simulink model "SoftManipulatorModel"  (R2019a)
settings: Solver=VariableStepAuto  StartTime=0.0  StopTime=100  FixedStep=0.01  RelTol=1e-3
undefined symbols (not defined in the file): d, dq_init, k, l, m, q_init
libraries: dspinverses x1
(part 2 of 2)

== matlab function SoftManipulatorModel/Controller/Coriolis Matrix ==
  data: q input; Cq output; dq input; m input; l input
function Cq = fcn(q, dq, m, l)

q1 = q(1);
q2 = q(2);
dq1 = dq(1);
dq2 = dq(2);
m1 = m(1);
m2 = m(2);
l1 = l(1);
l2 = l(2);

Cq = zeros(2,2);
% C111 = 0;
% C121 = 0;
% C221 = 0;
% C112 = 0;
% C222 = 0;
% tolerance = 1e-3;
% fake_zero = 1e-3;

% This equation got from Matlab symbolic calculation
% if abs(q1) < tolerance && abs(q2) > tolerance
%     C111 = 0;
%     C121 = -(m2*((l2*sin(conj(q2))*conj(l2)*(cos(q2) - 1))/(4*q2*conj(q2)) - ((l2*cos(q2))/(2*q2) - (l2*sin(q2))/(2*q2^2))*(conj(l1) + (sin(conj(q2))*conj(l2))/(2*conj(q2))) - (l1 + (l2*sin(q2))/(2*q2))*((cos(conj(q2))*conj(l2))/(2*conj(q2)) - (sin(conj(q2))*conj(l2))/(2*conj(q2)^2)) + (l2*conj(l2)*sin(q2)*(cos(conj(q2)) - 1))/(4*q2*conj(q2)) + (l2*conj(l2)*(cos(q2) - 1)*(cos(conj(q2)) - 1))/(4*q2*conj(q2)^2) + (l2*conj(l2)*(cos(q2) - 1)*(cos(conj(q2)) - 1))/(4*q2^2*conj(q2))))/2;
%     C221 = -m2*((l2*sin(q2)*(conj(l1) + (sin(conj(q2))*conj(l2))/(2*conj(q2))))/(2*q2^2) - (l2*cos(q2)*(conj(l1) + (sin(conj(q2))*conj(l2))/(2*conj(q2))))/(2*q2) - (l2*sin(q2)*((cos(conj(q2))*conj(l2))/(2*conj(q2)) - (sin(conj(q2))*conj(l2))/(2*conj(q2)^2)))/(2*q2) + (l2*sin(conj(q2))*conj(l2)*(cos(q2) - 1))/(4*q2*conj(q2)) + (l2*conj(l2)*sin(q2)*(cos(conj(q2)) - 1))/(4*q2*conj(q2)) + (l2*conj(l2)*(cos(q2) - 1)*(cos(conj(q2)) - 1))/(4*q2*conj(q2)^2) + (l2*conj(l2)*(cos(q2) - 1)*(cos(conj(q2)) - 1))/(4*q2^2*conj(q2)));
%     C112 = (m2*((l2*sin(conj(q2))*conj(l2)*(cos(q2) - 1))/(4*q2*conj(q2)) - ((l2*cos(q2))/(2*q2) - (l2*sin(q2))/(2*q2^2))*(conj(l1) + (sin(conj(q2))*conj(l2))/(2*conj(q2))) - (l1 + (l2*sin(q2))/(2*q2))*((cos(conj(q2))*conj(l2))/(2*conj(q2)) - (sin(conj(q2))*conj(l2))/(2*conj(q2)^2)) + (l2*conj(l2)*sin(q2)*(cos(conj(q2)) - 1))/(4*q2*conj(q2)) + (l2*conj(l2)*(cos(q2) - 1)*(cos(conj(q2)) - 1))/(4*q2*conj(q2)^2) + (l2*conj(l2)*(cos(q2) - 1)*(cos(conj(q2)) - 1))/(4*q2^2*conj(q2))))/2;
%     C222 = -(m2*((l2*sin(conj(q2))*conj(l2)*(cos(q2) - 1))/(4*q2*conj(q2)) + (l2*conj(l2)*sin(q2)*(cos(conj(q2)) - 1))/(4*q2*conj(q2)) + (l2*conj(l2)*(cos(q2) - 1)*(cos(conj(q2)) - 1))/(4*q2*conj(q2)^2) + (l2*conj(l2)*(cos(q2) - 1)*(cos(conj(q2)) - 1))/(4*q2^2*conj(q2)) - (l2*cos(conj(q2))*conj(l2)*sin(q2))/(4*q2*conj(q2)) - (l2*sin(conj(q2))*conj(l2)*cos(q2))/(4*q2*conj(q2)) + (l2*sin(conj(q2))*conj(l2)*sin(q2))/(4*q2*conj(q2)^2) + (l2*sin(conj(q2))*conj(l2)*sin(q2))/(4*q2^2*conj(q2))))/2;
% elseif abs(q1) < tolerance && abs(q2) < tolerance
%     C111 = 0;
%     C121 = 0;
%     C221 = 0;
%     C112 = 0;
%     C222 = 0;
% elseif abs(q1) > tolerance && abs(q2) < tolerance
%     C111 = m2*(((sin(conj(q1))*conj(l2))/2 - (conj(l1)*(cos(conj(q1)) - 1))/conj(q1))*((l2*cos(q1))/2 + (l1*sin(q1))/q1 + (l1*(cos(q1) - 1))/q1^2) + ((l2*sin(q1))/2 - (l1*(cos(q1) - 1))/q1)*((cos(conj(q1))*conj(l2))/2 + (sin(conj(q1))*conj(l1))/conj(q1) + (conj(l1)*(cos(conj(q1)) - 1))/conj(q1)^2) - ((cos(conj(q1))*conj(l2))/2 + (sin(conj(q1))*conj(l1))/conj(q1))*((l2*sin(q1))/2 - (l1*cos(q1))/q1 + (l1*sin(q1))/q1^2) - ((l2*cos(q1))/2 + (l1*sin(q1))/q1)*((sin(conj(q1))*conj(l2))/2 - (cos(conj(q1))*conj(l1))/conj(q1) + (sin(conj(q1))*conj(l1))/conj(q1)^2)) - m1*((l1*sin(conj(q1))*conj(l1)*(cos(q1) - 1))/(4*q1*conj(q1)) + (l1*conj(l1)*sin(q1)*(cos(conj(q1)) - 1))/(4*q1*conj(q1)) + (l1*conj(l1)*(cos(q1) - 1)*(cos(conj(q1)) - 1))/(4*q1*conj(q1)^2) + (l1*conj(l1)*(cos(q1) - 1)*(cos(conj(q1)) - 1))/(4*q1^2*conj(q1)) - (l1*cos(conj(q1))*conj(l1)*sin(q1))/(4*q1*conj(q1)) - (l1*sin(conj(q1))*conj(l1)*cos(q1))/(4*q1*conj(q1)) + (l1*sin(conj(q1))*conj(l1)*sin(q1))/(4*q1*conj(q1)^2) + (l1*sin(conj(q1))*conj(l1)*sin(q1))/(4*q1^2*conj(q1)));
%     C121 = 0;
%     C221 = 0;
%     C112 = m2*((cos(conj(q1))*conj(l2)*((l2*sin(q1))/2 - (l1*(cos(q1) - 1))/q1))/2 - (cos(conj(q1))*conj(l2)*((l2*sin(q1))/2 - (l1*cos(q1))/q1 + (l1*sin(q1))/q1^2))/2 + (sin(conj(q1))*conj(l2)*((l2*cos(q1))/2 + (l1*sin(q1))/q1 + (l1*(cos(q1) - 1))/q1^2))/2 - (sin(conj(q1))*conj(l2)*((l2*cos(q1))/2 + (l1*sin(q1))/q1))/2);
%     C222 = 0;
% elseif abs(q1) > tolerance && abs(q2) > tolerance
%     C111 = m2*(((l1*sin(q1))/q1 + (l2*cos(q1)*sin(q2))/(2*q2) + (l2*sin(q1)*(cos(q2) - 1))/(2*q2))*((cos(conj(q1))*conj(l1))/conj(q1) - (sin(conj(q1))*conj(l1))/conj(q1)^2 + (cos(conj(q1))*conj(l2)*(cos(conj(q2)) - 1))/(2*conj(q2)) - (sin(conj(q1))*sin(conj(q2))*conj(l2))/(2*conj(q2))) - ((conj(l1)*(cos(conj(q1)) - 1))/conj(q1) + (cos(conj(q1))*conj(l2)*(cos(conj(q2)) - 1))/(2*conj(q2)) - (sin(conj(q1))*sin(conj(q2))*conj(l2))/(2*conj(q2)))*((l1*sin(q1))/q1 + (l1*(cos(q1) - 1))/q1^2 + (l2*cos(q1)*sin(q2))/(2*q2) + (l2*sin(q1)*(cos(q2) - 1))/(2*q2)) - ((l1*(cos(q1) - 1))/q1 - (l2*sin(q1)*sin(q2))/(2*q2) + (l2*cos(q1)*(cos(q2) - 1))/(2*q2))*((sin(conj(q1))*conj(l1))/conj(q1) + (conj(l1)*(cos(conj(q1)) - 1))/conj(q1)^2 + (sin(conj(q1))*conj(l2)*(cos(conj(q2)) - 1))/(2*conj(q2)) + (cos(conj(q1))*sin(conj(q2))*conj(l2))/(2*conj(q2))) + ((sin(conj(q1))*conj(l1))/conj(q1) + (sin(conj(q1))*conj(l2)*(cos(conj(q2)) - 1))/(2*conj(q2)) + (cos(conj(q1))*sin(conj(q2))*conj(l2))/(2*conj(q2)))*((l1*cos(q1))/q1 - (l1*sin(q1))/q1^2 - (l2*sin(q1)*sin(q2))/(2*q2) + (l2*cos(q1)*(cos(q2) - 1))/(2*q2))) - m1*((l1*sin(conj(q1))*conj(l1)*(cos(q1) - 1))/(4*q1*conj(q1)) + (l1*conj(l1)*sin(q1)*(cos(conj(q1)) - 1))/(4*q1*conj(q1)) + (l1*conj(l1)*(cos(q1) - 1)*(cos(conj(q1)) - 1))/(4*q1*conj(q1)^2) + (l1*conj(l1)*(cos(q1) - 1)*(cos(conj(q1)) - 1))/(4*q1^2*conj(q1)) - (l1*cos(conj(q1))*conj(l1)*sin(q1))/(4*q1*conj(q1)) - (l1*sin(conj(q1))*conj(l1)*cos(q1))/(4*q1*conj(q1)) + (l1*sin(conj(q1))*conj(l1)*sin(q1))/(4*q1*conj(q1)^2) + (l1*sin(conj(q1))*conj(l1)*sin(q1))/(4*q1^2*conj(q1)));
%     C121 = -(m2*(((l1*sin(q1))/q1 + (l2*cos(q1)*sin(q2))/(2*q2) + (l2*sin(q1)*(cos(q2) - 1))/(2*q2))*((sin(conj(q1))*conj(l2)*(cos(conj(q2)) - 1))/(2*conj(q2)^2) - (cos(conj(q1))*cos(conj(q2))*conj(l2))/(2*conj(q2)) + (cos(conj(q1))*sin(conj(q2))*conj(l2))/(2*conj(q2)^2) + (sin(conj(q1))*sin(conj(q2))*conj(l2))/(2*conj(q2))) + ((sin(conj(q1))*conj(l1))/conj(q1) + (sin(conj(q1))*conj(l2)*(cos(conj(q2)) - 1))/(2*conj(q2)) + (cos(conj(q1))*sin(conj(q2))*conj(l2))/(2*conj(q2)))*((l2*cos(q1)*sin(q2))/(2*q2^2) - (l2*cos(q1)*cos(q2))/(2*q2) + (l2*sin(q1)*sin(q2))/(2*q2) + (l2*sin(q1)*(cos(q2) - 1))/(2*q2^2)) + ((l1*(cos(q1) - 1))/q1 - (l2*sin(q1)*sin(q2))/(2*q2) + (l2*cos(q1)*(cos(q2) - 1))/(2*q2))*((cos(conj(q1))*conj(l2)*(cos(conj(q2)) - 1))/(2*conj(q2)^2) + (cos(conj(q1))*sin(conj(q2))*conj(l2))/(2*conj(q2)) + (cos(conj(q2))*sin(conj(q1))*conj(l2))/(2*conj(q2)) - (sin(conj(q1))*sin(conj(q2))*conj(l2))/(2*conj(q2)^2)) + ((conj(l1)*(cos(conj(q1)) - 1))/conj(q1) + (cos(conj(q1))*conj(l2)*(cos(conj(q2)) - 1))/(2*conj(q2)) - (sin(conj(q1))*sin(conj(q2))*conj(l2))/(2*conj(q2)))*((l2*cos(q1)*sin(q2))/(2*q2) + (l2*cos(q2)*sin(q1))/(2*q2) - (l2*sin(q1)*sin(q2))/(2*q2^2) + (l2*cos(q1)*(cos(q2) - 1))/(2*q2^2))))/2;
%     C221 = -m2*(((l2*cos(q1)*sin(q2))/(2*q2) + (l2*sin(q1)*(cos(q2) - 1))/(2*q2))*((sin(conj(q1))*conj(l2)*(cos(conj(q2)) - 1))/(2*conj(q2)^2) - (cos(conj(q1))*cos(conj(q2))*conj(l2))/(2*conj(q2)) + (cos(conj(q1))*sin(conj(q2))*conj(l2))/(2*conj(q2)^2) + (sin(conj(q1))*sin(conj(q2))*conj(l2))/(2*conj(q2))) - ((l2*sin(q1)*sin(q2))/(2*q2) - (l2*cos(q1)*(cos(q2) - 1))/(2*q2))*((cos(conj(q1))*conj(l2)*(cos(conj(q2)) - 1))/(2*conj(q2)^2) + (cos(conj(q1))*sin(conj(q2))*conj(l2))/(2*conj(q2)) + (cos(conj(q2))*sin(conj(q1))*conj(l2))/(2*conj(q2)) - (sin(conj(q1))*sin(conj(q2))*conj(l2))/(2*conj(q2)^2)) + ((sin(conj(q1))*conj(l1))/conj(q1) + (sin(conj(q1))*conj(l2)*(cos(conj(q2)) - 1))/(2*conj(q2)) + (cos(conj(q1))*sin(conj(q2))*conj(l2))/(2*conj(q2)))*((l2*cos(q1)*sin(q2))/(2*q2^2) - (l2*cos(q1)*cos(q2))/(2*q2) + (l2*sin(q1)*sin(q2))/(2*q2) + (l2*sin(q1)*(cos(q2) - 1))/(2*q2^2)) + ((conj(l1)*(cos(conj(q1)) - 1))/conj(q1) + (cos(conj(q1))*conj(l2)*(cos(conj(q2)) - 1))/(2*conj(q2)) - (sin(conj(q1))*sin(conj(q2))*conj(l2))/(2*conj(q2)))*((l2*cos(q1)*sin(q2))/(2*q2) + (l2*cos(q2)*sin(q1))/(2*q2) - (l2*sin(q1)*sin(q2))/(2*q2^2) + (l2*cos(q1)*(cos(q2) - 1))/(2*q2^2)));
%     C112 = (m2*(((l1*sin(q1))/q1 + (l2*cos(q1)*sin(q2))/(2*q2) + (l2*sin(q1)*(cos(q2) - 1))/(2*q2))*((sin(conj(q1))*conj(l2)*(cos(conj(q2)) - 1))/(2*conj(q2)^2) - (cos(conj(q1))*cos(conj(q2))*conj(l2))/(2*conj(q2)) + (cos(conj(q1))*sin(conj(q2))*conj(l2))/(2*conj(q2)^2) + (sin(conj(q1))*sin(conj(q2))*conj(l2))/(2*conj(q2))) + ((sin(conj(q1))*conj(l1))/conj(q1) + (sin(conj(q1))*conj(l2)*(cos(conj(q2)) - 1))/(2*conj(q2)) + (cos(conj(q1))*sin(conj(q2))*conj(l2))/(2*conj(q2)))*((l2*cos(q1)*sin(q2))/(2*q2^2) - (l2*cos(q1)*cos(q2))/(2*q2) + (l2*sin(q1)*sin(q2))/(2*q2) + (l2*sin(q1)*(cos(q2) - 1))/(2*q2^2)) + ((l1*(cos(q1) - 1))/q1 - (l2*sin(q1)*sin(q2))/(2*q2) + (l2*cos(q1)*(cos(q2) - 1))/(2*q2))*((cos(conj(q1))*conj(l2)*(cos(conj(q2)) - 1))/(2*conj(q2)^2) + (cos(conj(q1))*sin(conj(q2))*conj(l2))/(2*conj(q2)) + (cos(conj(q2))*sin(conj(q1))*conj(l2))/(2*conj(q2)) - (sin(conj(q1))*sin(conj(q2))*conj(l2))/(2*conj(q2)^2)) + ((conj(l1)*(cos(conj(q1)) - 1))/conj(q1) + (cos(conj(q1))*conj(l2)*(cos(conj(q2)) - 1))/(2*conj(q2)) - (sin(conj(q1))*sin(conj(q2))*conj(l2))/(2*conj(q2)))*((l2*cos(q1)*sin(q2))/(2*q2) + (l2*cos(q2)*sin(q1))/(2*q2) - (l2*sin(q1)*sin(q2))/(2*q2^2) + (l2*cos(q1)*(cos(q2) - 1))/(2*q2^2))))/2 - m2*(((sin(conj(q1))*conj(l2)*(cos(conj(q2)) - 1))/(2*conj(q2)) + (cos(conj(q1))*sin(conj(q2))*conj(l2))/(2*conj(q2)))*((l1*(cos(q1) - 1))/q1 - (l2*sin(q1)*sin(q2))/(2*q2) + (l2*cos(q1)*(cos(q2) - 1))/(2*q2)) - ((sin(conj(q1))*conj(l2)*(cos(conj(q2)) - 1))/(2*conj(q2)) + (cos(conj(q1))*sin(conj(q2))*conj(l2))/(2*conj(q2)))*((l1*cos(q1))/q1 - (l1*sin(q1))/q1^2 - (l2*sin(q1)*sin(q2))/(2*q2) + (l2*cos(q1)*(cos(q2) - 1))/(2*q2)) + ((cos(conj(q1))*conj(l2)*(cos(conj(q2)) - 1))/(2*conj(q2)) - (sin(conj(q1))*sin(conj(q2))*conj(l2))/(2*conj(q2)))*((l1*sin(q1))/q1 + (l1*(cos(q1) - 1))/q1^2 + (l2*cos(q1)*sin(q2))/(2*q2) + (l2*sin(q1)*(cos(q2) - 1))/(2*q2)) - ((cos(conj(q1))*conj(l2)*(cos(conj(q2)) - 1))/(2*conj(q2)) - (sin(conj(q1))*sin(conj(q2))*conj(l2))/(2*conj(q2)))*((l1*sin(q1))/q1 + (l2*cos(q1)*sin(q2))/(2*q2) + (l2*sin(q1)*(cos(q2) - 1))/(2*q2)));
%     C222 = -(m2*(((l2*cos(q1)*sin(q2))/(2*q2) + (l2*sin(q1)*(cos(q2) - 1))/(2*q2))*((sin(conj(q1))*conj(l2)*(cos(conj(q2)) - 1))/(2*conj(q2)^2) - (cos(conj(q1))*cos(conj(q2))*conj(l2))/(2*conj(q2)) + (cos(conj(q1))*sin(conj(q2))*conj(l2))/(2*conj(q2)^2) + (sin(conj(q1))*sin(conj(q2))*conj(l2))/(2*conj(q2))) - ((l2*sin(q1)*sin(q2))/(2*q2) - (l2*cos(q1)*(cos(q2) - 1))/(2*q2))*((cos(conj(q1))*conj(l2)*(cos(conj(q2)) - 1))/(2*conj(q2)^2) + (cos(conj(q1))*sin(conj(q2))*conj(l2))/(2*conj(q2)) + (cos(conj(q2))*sin(conj(q1))*conj(l2))/(2*conj(q2)) - (sin(conj(q1))*sin(conj(q2))*conj(l2))/(2*conj(q2)^2)) + ((cos(conj(q1))*conj(l2)*(cos(conj(q2)) - 1))/(2*conj(q2)) - (sin(conj(q1))*sin(conj(q2))*conj(l2))/(2*conj(q2)))*((l2*cos(q1)*sin(q2))/(2*q2) + (l2*cos(q2)*sin(q1))/(2*q2) - (l2*sin(q1)*sin(q2))/(2*q2^2) + (l2*cos(q1)*(cos(q2) - 1))/(2*q2^2)) + ((sin(conj(q1))*conj(l2)*(cos(conj(q2)) - 1))/(2*conj(q2)) + (cos(conj(q1))*sin(conj(q2))*conj(l2))/(2*conj(q2)))*((l2*cos(q1)*sin(q2))/(2*q2^2) - (l2*cos(q1)*cos(q2))/(2*q2) + (l2*sin(q1)*sin(q2))/(2*q2) + (l2*sin(q1)*(cos(q2) - 1))/(2*q2^2))))/2;
% end

% if abs(q1) < tolerance && abs(q2) > tolerance
%     if q1 < 0
%         q1 = -fake_zero;
%     else
%         q1 = fake_zero;
%     end
% elseif abs(q1) < tolerance && abs(q2) < tolerance
%     if q1 < 0
%         q1 = -fake_zero;
%     else
%         q1 = fake_zero;
%     end
%     
%     if q2 < 0
%         q2 = -fake_zero;
%     else
%         q2 = fake_zero;
%     end
% elseif abs(q1) > tolerance && abs(q2) < tolerance
%     if q2 < 0
%         q2 = -fake_zero;
%     else
%         q2 = fake_zero;
%     end
% end

C111 = m2*(((l1*sin(q1))/q1 + (l2*cos(q1)*sin(q2))/(2*q2) + (l2*sin(q1)*(cos(q2) - 1))/(2*q2))*((cos(conj(q1))*conj(l1))/conj(q1) - (sin(conj(q1))*conj(l1))/conj(q1)^2 + (cos(conj(q1))*conj(l2)*(cos(conj(q2)) - 1))/(2*conj(q2)) - (sin(conj(q1))*sin(conj(q2))*conj(l2))/(2*conj(q2))) - ((conj(l1)*(cos(conj(q1)) - 1))/conj(q1) + (cos(conj(q1))*conj(l2)*(cos(conj(q2)) - 1))/(2*conj(q2)) - (sin(conj(q1))*sin(conj(q2))*conj(l2))/(2*conj(q2)))*((l1*sin(q1))/q1 + (l1*(cos(q1) - 1))/q1^2 + (l2*cos(q1)*sin(q2))/(2*q2) + (l2*sin(q1)*(cos(q2) - 1))/(2*q2)) - ((l1*(cos(q1) - 1))/q1 - (l2*sin(q1)*sin(q2))/(2*q2) + (l2*cos(q1)*(cos(q2) - 1))/(2*q2))*((sin(conj(q1))*conj(l1))/conj(q1) + (conj(l1)*(cos(conj(q1)) - 1))/conj(q1)^2 + (sin(conj(q1))*conj(l2)*(cos(conj(q2)) - 1))/(2*conj(q2)) + (cos(conj(q1))*sin(conj(q2))*conj(l2))/(2*conj(q2))) + ((sin(conj(q1))*conj(l1))/conj(q1) + (sin(conj(q1))*conj(l2)*(cos(conj(q2)) - 1))/(2*conj(q2)) + (cos(conj(q1))*sin(conj(q2))*conj(l2))/(2*conj(q2)))*((l1*cos(q1))/q1 - (l1*sin(q1))/q1^2 - (l2*sin(q1)*sin(q2))/(2*q2) + (l2*cos(q1)*(cos(q2) - 1))/(2*q2))) - m1*((l1*sin(conj(q1))*conj(l1)*(cos(q1) - 1))/(4*q1*conj(q1)) + (l1*conj(l1)*sin(q1)*(cos(conj(q1)) - 1))/(4*q1*conj(q1)) + (l1*conj(l1)*(cos(q1) - 1)*(cos(conj(q1)) - 1))/(4*q1*conj(q1)^2) + (l1*conj(l1)*(cos(q1) - 1)*(cos(conj(q1)) - 1))/(4*q1^2*conj(q1)) - (l1*cos(conj(q1))*conj(l1)*sin(q1))/(4*q1*conj(q1)) - (l1*sin(conj(q1))*conj(l1)*cos(q1))/(4*q1*conj(q1)) + (l1*sin(conj(q1))*conj(l1)*sin(q1))/(4*q1*conj(q1)^2) + (l1*sin(conj(q1))*conj(l1)*sin(q1))/(4*q1^2*conj(q1)));
C121 = -(m2*(((l1*sin(q1))/q1 + (l2*cos(q1)*sin(q2))/(2*q2) + (l2*sin(q1)*(cos(q2) - 1))/(2*q2))*((sin(conj(q1))*conj(l2)*(cos(conj(q2)) - 1))/(2*conj(q2)^2) - (cos(conj(q1))*cos(conj(q2))*conj(l2))/(2*conj(q2)) + (cos(conj(q1))*sin(conj(q2))*conj(l2))/(2*conj(q2)^2) + (sin(conj(q1))*sin(conj(q2))*conj(l2))/(2*conj(q2))) + ((sin(conj(q1))*conj(l1))/conj(q1) + (sin(conj(q1))*conj(l2)*(cos(conj(q2)) - 1))/(2*conj(q2)) + (cos(conj(q1))*sin(conj(q2))*conj(l2))/(2*conj(q2)))*((l2*cos(q1)*sin(q2))/(2*q2^2) - (l2*cos(q1)*cos(q2))/(2*q2) + (l2*sin(q1)*sin(q2))/(2*q2) + (l2*sin(q1)*(cos(q2) - 1))/(2*q2^2)) + ((l1*(cos(q1) - 1))/q1 - (l2*sin(q1)*sin(q2))/(2*q2) + (l2*cos(q1)*(cos(q2) - 1))/(2*q2))*((cos(conj(q1))*conj(l2)*(cos(conj(q2)) - 1))/(2*conj(q2)^2) + (cos(conj(q1))*sin(conj(q2))*conj(l2))/(2*conj(q2)) + (cos(conj(q2))*sin(conj(q1))*conj(l2))/(2*conj(q2)) - (sin(conj(q1))*sin(conj(q2))*conj(l2))/(2*conj(q2)^2)) + ((conj(l1)*(cos(conj(q1)) - 1))/conj(q1) + (cos(conj(q1))*conj(l2)*(cos(conj(q2)) - 1))/(2*conj(q2)) - (sin(conj(q1))*sin(conj(q2))*conj(l2))/(2*conj(q2)))*((l2*cos(q1)*sin(q2))/(2*q2) + (l2*cos(q2)*sin(q1))/(2*q2) - (l2*sin(q1)*sin(q2))/(2*q2^2) + (l2*cos(q1)*(cos(q2) - 1))/(2*q2^2))))/2;
C221 = -m2*(((l2*cos(q1)*sin(q2))/(2*q2) + (l2*sin(q1)*(cos(q2) - 1))/(2*q2))*((sin(conj(q1))*conj(l2)*(cos(conj(q2)) - 1))/(2*conj(q2)^2) - (cos(conj(q1))*cos(conj(q2))*conj(l2))/(2*conj(q2)) + (cos(conj(q1))*sin(conj(q2))*conj(l2))/(2*conj(q2)^2) + (sin(conj(q1))*sin(conj(q2))*conj(l2))/(2*conj(q2))) - ((l2*sin(q1)*sin(q2))/(2*q2) - (l2*cos(q1)*(cos(q2) - 1))/(2*q2))*((cos(conj(q1))*conj(l2)*(cos(conj(q2)) - 1))/(2*conj(q2)^2) + (cos(conj(q1))*sin(conj(q2))*conj(l2))/(2*conj(q2)) + (cos(conj(q2))*sin(conj(q1))*conj(l2))/(2*conj(q2)) - (sin(conj(q1))*sin(conj(q2))*conj(l2))/(2*conj(q2)^2)) + ((sin(conj(q1))*conj(l1))/conj(q1) + (sin(conj(q1))*conj(l2)*(cos(conj(q2)) - 1))/(2*conj(q2)) + (cos(conj(q1))*sin(conj(q2))*conj(l2))/(2*conj(q2)))*((l2*cos(q1)*sin(q2))/(2*q2^2) - (l2*cos(q1)*cos(q2))/(2*q2) + (l2*sin(q1)*sin(q2))/(2*q2) + (l2*sin(q1)*(cos(q2) - 1))/(2*q2^2)) + ((conj(l1)*(cos(conj(q1)) - 1))/conj(q1) + (cos(conj(q1))*conj(l2)*(cos(conj(q2)) - 1))/(2*conj(q2)) - (sin(conj(q1))*sin(conj(q2))*conj(l2))/(2*conj(q2)))*((l2*cos(q1)*sin(q2))/(2*q2) + (l2*cos(q2)*sin(q1))/(2*q2) - (l2*sin(q1)*sin(q2))/(2*q2^2) + (l2*cos(q1)*(cos(q2) - 1))/(2*q2^2)));
C112 = (m2*(((l1*sin(q1))/q1 + (l2*cos(q1)*sin(q2))/(2*q2) + (l2*sin(q1)*(cos(q2) - 1))/(2*q2))*((sin(conj(q1))*conj(l2)*(cos(conj(q2)) - 1))/(2*conj(q2)^2) - (cos(conj(q1))*cos(conj(q2))*conj(l2))/(2*conj(q2)) + (cos(conj(q1))*sin(conj(q2))*conj(l2))/(2*conj(q2)^2) + (sin(conj(q1))*sin(conj(q2))*conj(l2))/(2*conj(q2))) + ((sin(conj(q1))*conj(l1))/conj(q1) + (sin(conj(q1))*conj(l2)*(cos(conj(q2)) - 1))/(2*conj(q2)) + (cos(conj(q1))*sin(conj(q2))*conj(l2))/(2*conj(q2)))*((l2*cos(q1)*sin(q2))/(2*q2^2) - (l2*cos(q1)*cos(q2))/(2*q2) + (l2*sin(q1)*sin(q2))/(2*q2) + (l2*sin(q1)*(cos(q2) - 1))/(2*q2^2)) + ((l1*(cos(q1) - 1))/q1 - (l2*sin(q1)*sin(q2))/(2*q2) + (l2*cos(q1)*(cos(q2) - 1))/(2*q2))*((cos(conj(q1))*conj(l2)*(cos(conj(q2)) - 1))/(2*conj(q2)^2) + (cos(conj(q1))*sin(conj(q2))*conj(l2))/(2*conj(q2)) + (cos(conj(q2))*sin(conj(q1))*conj(l2))/(2*conj(q2)) - (sin(conj(q1))*sin(conj(q2))*conj(l2))/(2*conj(q2)^2)) + ((conj(l1)*(cos(conj(q1)) - 1))/conj(q1) + (cos(conj(q1))*conj(l2)*(cos(conj(q2)) - 1))/(2*conj(q2)) - (sin(conj(q1))*sin(conj(q2))*conj(l2))/(2*conj(q2)))*((l2*cos(q1)*sin(q2))/(2*q2) + (l2*cos(q2)*sin(q1))/(2*q2) - (l2*sin(q1)*sin(q2))/(2*q2^2) + (l2*cos(q1)*(cos(q2) - 1))/(2*q2^2))))/2 - m2*(((sin(conj(q1))*conj(l2)*(cos(conj(q2)) - 1))/(2*conj(q2)) + (cos(conj(q1))*sin(conj(q2))*conj(l2))/(2*conj(q2)))*((l1*(cos(q1) - 1))/q1 - (l2*sin(q1)*sin(q2))/(2*q2) + (l2*cos(q1)*(cos(q2) - 1))/(2*q2)) - ((sin(conj(q1))*conj(l2)*(cos(conj(q2)) - 1))/(2*conj(q2)) + (cos(conj(q1))*sin(conj(q2))*conj(l2))/(2*conj(q2)))*((l1*cos(q1))/q1 - (l1*sin(q1))/q1^2 - (l2*sin(q1)*sin(q2))/(2*q2) + (l2*cos(q1)*(cos(q2) - 1))/(2*q2)) + ((cos(conj(q1))*conj(l2)*(cos(conj(q2)) - 1))/(2*conj(q2)) - (sin(conj(q1))*sin(conj(q2))*conj(l2))/(2*conj(q2)))*((l1*sin(q1))/q1 + (l1*(cos(q1) - 1))/q1^2 + (l2*cos(q1)*sin(q2))/(2*q2) + (l2*sin(q1)*(cos(q2) - 1))/(2*q2)) - ((cos(conj(q1))*conj(l2)*(cos(conj(q2)) - 1))/(2*conj(q2)) - (sin(conj(q1))*sin(conj(q2))*conj(l2))/(2*conj(q2)))*((l1*sin(q1))/q1 + (l2*cos(q1)*sin(q2))/(2*q2) + (l2*sin(q1)*(cos(q2) - 1))/(2*q2)));
C222 = -(m2*(((l2*cos(q1)*sin(q2))/(2*q2) + (l2*sin(q1)*(cos(q2) - 1))/(2*q2))*((sin(conj(q1))*conj(l2)*(cos(conj(q2)) - 1))/(2*conj(q2)^2) - (cos(conj(q1))*cos(conj(q2))*conj(l2))/(2*conj(q2)) + (cos(conj(q1))*sin(conj(q2))*conj(l2))/(2*conj(q2)^2) + (sin(conj(q1))*sin(conj(q2))*conj(l2))/(2*conj(q2))) - ((l2*sin(q1)*sin(q2))/(2*q2) - (l2*cos(q1)*(cos(q2) - 1))/(2*q2))*((cos(conj(q1))*conj(l2)*(cos(conj(q2)) - 1))/(2*conj(q2)^2) + (cos(conj(q1))*sin(conj(q2))*conj(l2))/(2*conj(q2)) + (cos(conj(q2))*sin(conj(q1))*conj(l2))/(2*conj(q2)) - (sin(conj(q1))*sin(conj(q2))*conj(l2))/(2*conj(q2)^2)) + ((cos(conj(q1))*conj(l2)*(cos(conj(q2)) - 1))/(2*conj(q2)) - (sin(conj(q1))*sin(conj(q2))*conj(l2))/(2*conj(q2)))*((l2*cos(q1)*sin(q2))/(2*q2) + (l2*cos(q2)*sin(q1))/(2*q2) - (l2*sin(q1)*sin(q2))/(2*q2^2) + (l2*cos(q1)*(cos(q2) - 1))/(2*q2^2)) + ((sin(conj(q1))*conj(l2)*(cos(conj(q2)) - 1))/(2*conj(q2)) + (cos(conj(q1))*sin(conj(q2))*conj(l2))/(2*conj(q2)))*((l2*cos(q1)*sin(q2))/(2*q2^2) - (l2*cos(q1)*cos(q2))/(2*q2) + (l2*sin(q1)*sin(q2))/(2*q2) + (l2*sin(q1)*(cos(q2) - 1))/(2*q2^2))))/2;

Cq(1,1) = C111 * dq1;
Cq(1,2) = 2 * C121 * dq1 + C221 * dq2;
Cq(2,1) = C112 * dq1;
Cq(2,2) = C222 * dq2;

% for i = 1:2
%     for j = 1:2
%         if Cq(i,j) < tolerance
%             Cq(i,j) = 0;
%         end
%     end
% end

== matlab function SoftManipulatorModel/Controller/Potential Matrix ==
  data: q input; Gq output; m input; l input; g input
function Gq = fcn(q, m, l, g)

q1 = q(1);
q2 = q(2);
m1 = m(1);
m2 = m(2);
l1 = l(1);
l2 = l(2);

Gq = zeros(2,1);
% error_toler = 1e-3;

% This equation got from Matlab symbolic calculation
% if abs(q1) < error_toler && abs(q2) > error_toler
%     Gq(1,1) = 0;
%     Gq(2,1) = (g*l2*m2*sin(q2))/(2*q2) + (g*l2*m2*(cos(q2) - 1))/(2*q2^2);
% elseif abs(q1) < error_toler && abs(q2) < error_toler
%     Gq(1,1) = 0;
%     Gq(2,1) = 0;
% elseif abs(q1) > error_toler && abs(q2) < error_toler
%     Gq(1,1) = g*m2*((l2*cos(q1))/2 + (l1*sin(q1))/q1 + (l1*(cos(q1) - 1))/q1^2) + (g*l1*m1*sin(q1))/(2*q1) + (g*l1*m1*(cos(q1) - 1))/(2*q1^2);
%     Gq(2,1) = 0;
% elseif abs(q1) > error_toler && abs(q2) > error_toler
%     Gq(1,1) = (l1*sin(q1))/q1 + (l1*(cos(q1) - 1))/q1^2 + (l2*sin(q1)*(cos(q2) - 1))/(2*q2) + (g*l1*m1*sin(q1))/(2*q1) + (g*l1*m1*(cos(q1) - 1))/(2*q1^2) + (g*l2*m2*cos(q1)*sin(q2))/(2*q2);
%     Gq(2,1) = (l2*cos(q1)*sin(q2))/(2*q2) + (l2*cos(q1)*(cos(q2) - 1))/(2*q2^2) + (g*l2*m2*cos(q2)*sin(q1))/(2*q2) - (g*l2*m2*sin(q1)*sin(q2))/(2*q2^2);
% end

% if abs(q1) < error_toler && abs(q2) > error_toler
%     if q1 < 0
%         q1 = -error_toler;
%     else
%         q1 = error_toler;
%     end
% elseif abs(q1) < error_toler && abs(q2) < error_toler
%     if q1 < 0
%         q1 = -error_toler;
%     else
%         q1 = error_toler;
%     end
%     
%     if q2 < 0
%         q2 = -error_toler;
%     else
%         q2 = error_toler;
%     end
% elseif abs(q1) > error_toler && abs(q2) < error_toler
%     if q2 < 0
%         q2 = -error_toler;
%     else
%         q2 = error_toler;
%     end
% end

% Gq(1,1) = (l1*sin(q1))/q1 + (l1*(cos(q1) - 1))/q1^2 + (l2*sin(q1)*(cos(q2) - 1))/(2*q2) + (g*l1*m1*sin(q1))/(2*q1) + (g*l1*m1*(cos(q1) - 1))/(2*q1^2) + (g*l2*m2*cos(q1)*sin(q2))/(2*q2);
% Gq(2,1) = (l2*cos(q1)*sin(q2))/(2*q2) + (l2*cos(q1)*(cos(q2) - 1))/(2*q2^2) + (g*l2*m2*cos(q2)*sin(q1))/(2*q2) - (g*l2*m2*sin(q1)*sin(q2))/(2*q2^2);

Gq = [0; 0];

== matlab function SoftManipulatorModel/Controller/Elastic Term ==
  data: k input; K output
function K = fcn(k)

K = [k(1) 0; 0 k(2)];

== matlab function SoftManipulatorModel/Controller/ Dissipative Term ==
  data: d input; D output
function D = fcn(d)

D = [d(1) 0; 0 d(2)];
